simulink library "tf_sensor"  (R2026a)
settings: Solver=VariableStepAuto
libraries: nesl_utility x6, sm_lib x1
settings Model: Creator=th12-dv  LastModifiedBy=th12-dv

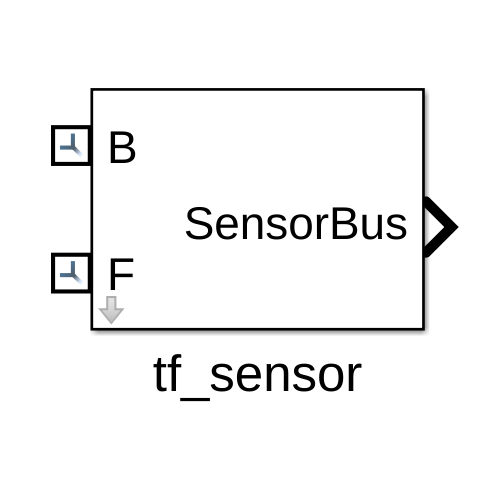
[thumbnail: Simulink's stored preview of the top-level diagram]
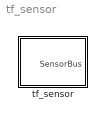
== system tf_sensor ==
  tf_sensor : Subsystem  mask(Transform Sensor with Bus Output){MeasurementFrame=World, RotationSequence=XYZ}
      mask prompts: MeasurementFrame "Measurement frame"; RotationSequence "Angle rotation sequence"
      mask help: Measures the transform between base frame B and follower frame F. Outputs a bus: Rotation (Angle, Omega, Alpha) and Translation (Pos, Vel, Acc).
      mask TypeOptions MeasurementFrame: Transform Sensor/MeasurementFrame
      mask TypeOptions RotationSequence: Transform Sensor/RotationSequence

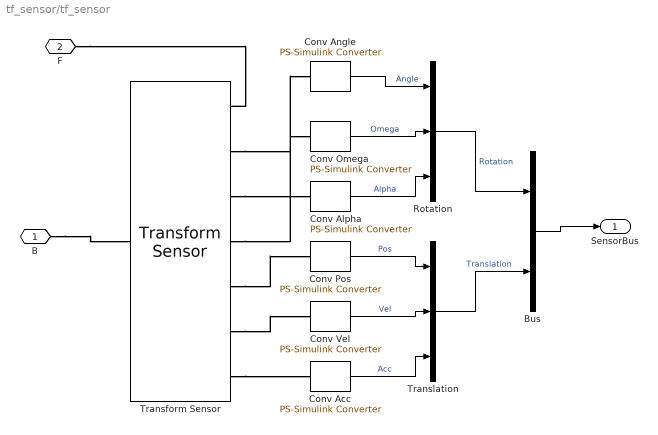
== system tf_sensor/tf_sensor ==
  Bus : BusCreator  Inputs=2
  Conv Acc : nesl_utility/PS-Simulink Converter  PhysicalDomain=network_engine_domain  SubClassName=ps_output  LeftPortType=input  RightPortType=output  PseudoPeriodic=off  Frequencies=[]  VectorFormat=inherit  Unit=m/s^2  AffineConversion=off
  Conv Alpha : nesl_utility/PS-Simulink Converter  PhysicalDomain=network_engine_domain  SubClassName=ps_output  LeftPortType=input  RightPortType=output  PseudoPeriodic=off  Frequencies=[]  VectorFormat=inherit  Unit=rad/s^2  AffineConversion=off
  Conv Angle : nesl_utility/PS-Simulink Converter  PhysicalDomain=network_engine_domain  SubClassName=ps_output  LeftPortType=input  RightPortType=output  PseudoPeriodic=off  Frequencies=[]  VectorFormat=inherit  Unit=rad  AffineConversion=off
  Conv Omega : nesl_utility/PS-Simulink Converter  PhysicalDomain=network_engine_domain  SubClassName=ps_output  LeftPortType=input  RightPortType=output  PseudoPeriodic=off  Frequencies=[]  VectorFormat=inherit  Unit=rad/s  AffineConversion=off
  Conv Pos : nesl_utility/PS-Simulink Converter  PhysicalDomain=network_engine_domain  SubClassName=ps_output  LeftPortType=input  RightPortType=output  PseudoPeriodic=off  Frequencies=[]  VectorFormat=inherit  Unit=m  AffineConversion=off
  Conv Vel : nesl_utility/PS-Simulink Converter  PhysicalDomain=network_engine_domain  SubClassName=ps_output  LeftPortType=input  RightPortType=output  PseudoPeriodic=off  Frequencies=[]  VectorFormat=inherit  Unit=m/s  AffineConversion=off
  Rotation : BusCreator  Inputs=3
  Transform Sensor : sm_lib/Frames and Transforms/Transform Sensor  MeasurementFrame=World  RotationSequence=XYZ  SenseAngle=off  SenseAxis=off  SenseQ=off  SenseR=off  SenseRotationSequence=on  SenseOmegaX=off  SenseOmegaY=off  SenseOmegaZ=off  SenseOmega=on  SenseQDot=off  SenseRDot=off  SenseRotationSequenceDot=off  SenseAlphaX=off  SenseAlphaY=off  SenseAlphaZ=off  SenseAlpha=on  SenseQDDot=off  SenseRDDot=off  SenseX=off  SenseY=off  SenseZ=off  SenseXYZ=on  SenseRad=off  SenseAzim=off  SenseDist=off  SenseInc=off  SenseXDot=off  SenseYDot=off  SenseZDot=off  SenseXYZDot=on  SenseRadDot=off  SenseAzimDot=off  SenseDistDot=off  SenseIncDot=off  SenseXDDot=off  SenseYDDot=off  SenseZDDot=off  SenseXYZDDot=on  SenseRadDDot=off  SenseAzimDDot=off  SenseDistDDot=off  SenseIncDDot=off
  Translation : BusCreator  Inputs=3
  B : PMIOPort  Side=Left
  F : PMIOPort  Port=2  Side=Left
  SensorBus : Outport
  wires:
  Conv Angle/1 -> Rotation/1  "Angle"
  Conv Omega/1 -> Rotation/2  "Omega"
  Conv Alpha/1 -> Rotation/3  "Alpha"
  Conv Pos/1 -> Translation/1  "Pos"
  Conv Vel/1 -> Translation/2  "Vel"
  Conv Acc/1 -> Translation/3  "Acc"
  Rotation/1 -> Bus/1  "Rotation"
  Translation/1 -> Bus/2  "Translation"
  Bus/1 -> SensorBus/1
  connections:
  B/RConn1 -- Transform Sensor/LConn1
  F/RConn1 -- Transform Sensor/RConn1
  Transform Sensor/RConn2 -- Conv Angle/LConn1
  Transform Sensor/RConn3 -- Conv Omega/LConn1
  Transform Sensor/RConn4 -- Conv Alpha/LConn1
  Transform Sensor/RConn5 -- Conv Pos/LConn1
  Transform Sensor/RConn6 -- Conv Vel/LConn1
  Transform Sensor/RConn7 -- Conv Acc/LConn1
